simulink model "sg_2d_fir"  (Simulink 7.6)
settings: Solver=ode45  StartTime=0.0  StopTime=1600.0  RelTol=1e-3
undefined symbols (not defined in the file): gcbh, xlBlockLoadCallback, xlGetNormalizedPeriod, xlipgetpartsetting
libraries: xbsIndex_r4 x311, dspsrcs4 x6
(part 4 of 4)

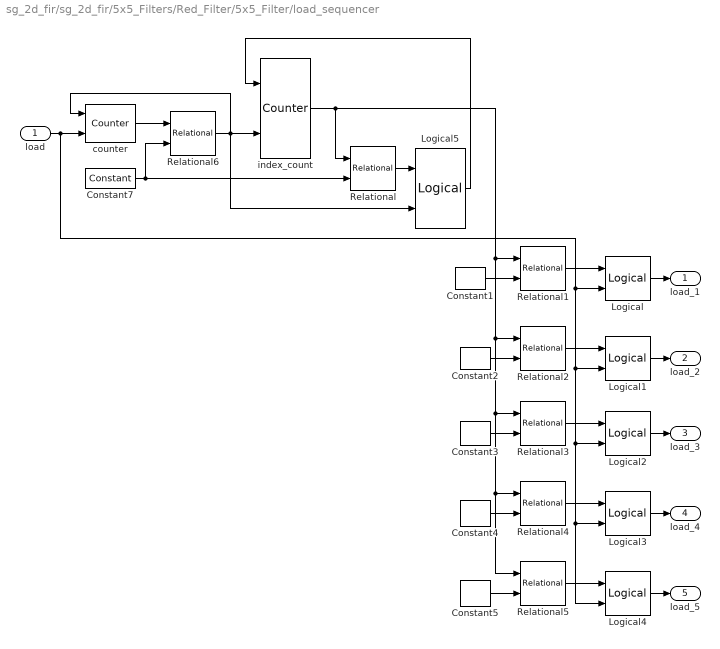
== system sg_2d_fir/sg_2d_fir/5x5_Filters/Red_Filter/5x5_Filter/load_sequencer ==
  load : Inport
  Constant1 : xbsIndex_r4/Constant  const=0  gui_display_data_type=Fixed-point  arith_type=Unsigned  n_bits=ceil(log2(num_coef))  bin_pt=0  preci_type=Single  exp_width=8  frac_width=24  explicit_period=off  period=1  equ=P=C  opselect=C  inp2=PCIN>>17  opr=+  inp1=P  carry=CIN  dbl_ovrd=off  block_type=constant
      settings: block_version=VER_STRING_GOES_HERE
  Constant2 : xbsIndex_r4/Constant  const=1  gui_display_data_type=Fixed-point  arith_type=Unsigned  n_bits=ceil(log2(num_coef))  bin_pt=0  preci_type=Single  exp_width=8  frac_width=24  explicit_period=off  period=1  equ=P=C  opselect=C  inp2=PCIN>>17  opr=+  inp1=P  carry=CIN  dbl_ovrd=off  block_type=constant
      settings: block_version=VER_STRING_GOES_HERE
  Constant3 : xbsIndex_r4/Constant  const=2  gui_display_data_type=Fixed-point  arith_type=Unsigned  n_bits=ceil(log2(num_coef))  bin_pt=0  preci_type=Single  exp_width=8  frac_width=24  explicit_period=off  period=1  equ=P=C  opselect=C  inp2=PCIN>>17  opr=+  inp1=P  carry=CIN  dbl_ovrd=off  block_type=constant
      settings: block_version=VER_STRING_GOES_HERE
  Constant4 : xbsIndex_r4/Constant  const=3  gui_display_data_type=Fixed-point  arith_type=Unsigned  n_bits=ceil(log2(num_coef))  bin_pt=0  preci_type=Single  exp_width=8  frac_width=24  explicit_period=off  period=1  equ=P=C  opselect=C  inp2=PCIN>>17  opr=+  inp1=P  carry=CIN  dbl_ovrd=off  block_type=constant
      settings: block_version=VER_STRING_GOES_HERE
  Constant5 : xbsIndex_r4/Constant  const=4  gui_display_data_type=Fixed-point  arith_type=Unsigned  n_bits=ceil(log2(num_coef))  bin_pt=0  preci_type=Single  exp_width=8  frac_width=24  explicit_period=off  period=1  equ=P=C  opselect=C  inp2=PCIN>>17  opr=+  inp1=P  carry=CIN  dbl_ovrd=off  block_type=constant
      settings: block_version=VER_STRING_GOES_HERE
  Constant7 : xbsIndex_r4/Constant  const=num_coef-1  gui_display_data_type=Fixed-point  arith_type=Unsigned  n_bits=ceil(log2(num_coef))  bin_pt=0  preci_type=Single  exp_width=8  frac_width=24  explicit_period=off  period=1  equ=P=C  opselect=C  inp2=PCIN>>17  opr=+  inp1=P  carry=CIN  dbl_ovrd=off  block_type=constant
      settings: block_version=VER_STRING_GOES_HERE
  Logical{,1..5} (6 alike) : xbsIndex_r4/Logical  logical_function=AND  inputs=2  en=off  latency=0  precision=Full  arith_type=Unsigned  n_bits=8  bin_pt=2  align_bp=on  dbl_ovrd=off  block_type=logical
      settings: xl_area=[0, 0, 0, 0, 0, 0, 0]  block_version=VER_STRING_GOES_HERE
  Relational{,1..6} (7 alike) : xbsIndex_r4/Relational  mode=a=b  en=off  latency=0  dbl_ovrd=off  block_type=relational
      settings: xl_area=[0, 0, 0, 0, 0, 0, 0]  block_version=VER_STRING_GOES_HERE
  counter : xbsIndex_r4/Counter  cnt_type=Count Limited  cnt_to=num_coef-1  operation=Up  start_count=0  cnt_by_val=1  arith_type=Unsigned  n_bits=ceil(log2(num_coef))  bin_pt=0  load_pin=off  rst=on  en=on  explicit_period=on  period=1  dbl_ovrd=off  use_behavioral_HDL=off  implementation=Fabric  use_rpm=off  block_type=counter
      settings: xl_area=[0, 0, 0, 0, 0, 0, 0]  block_version=VER_STRING_GOES_HERE
  index_count : xbsIndex_r4/Counter  cnt_type=Count Limited  cnt_to=num_coef-1  operation=Up  start_count=0  cnt_by_val=1  arith_type=Unsigned  n_bits=ceil(log2(num_coef))  bin_pt=0  load_pin=off  rst=on  en=on  explicit_period=on  period=1  dbl_ovrd=off  use_behavioral_HDL=off  implementation=Fabric  use_rpm=off  block_type=counter
      settings: infoedit="Configurable up, down and up/down counter.<P><P>Hardware notes: Free running counters are the least expensive in hardware.  A count limited counter is implemented by combining a counter with a comparator."  xl_area=[0, 0, 0, 0, 0, 0, 0]  block_version=VER_STRING_GOES_HERE
  load_1 : Outport
  load_2 : Outport  Port=2
  load_3 : Outport  Port=3
  load_4 : Outport  Port=4
  load_5 : Outport  Port=5
  wires:
  Constant1/1 -> Relational1/2
  Relational1/1 -> Logical/1
  Logical/1 -> load_1/1
  Constant2/1 -> Relational2/2
  Logical1/1 -> load_2/1
  Relational2/1 -> Logical1/1
  Constant3/1 -> Relational3/2
  Logical2/1 -> load_3/1
  Relational3/1 -> Logical2/1
  Constant4/1 -> Relational4/2
  Logical3/1 -> load_4/1
  Relational4/1 -> Logical3/1
  Constant5/1 -> Relational5/2
  Logical4/1 -> load_5/1
  Relational5/1 -> Logical4/1
  load/1 -> counter/2, Logical/2, Logical1/2, Logical2/2, Logical3/2, Logical4/2
  counter/1 -> Relational6/1
  Constant7/1 -> Relational6/2, Relational/2
  Relational6/1 -> index_count/2, counter/1, Logical5/2
  index_count/1 -> Relational/1, Relational1/1, Relational2/1, Relational3/1, Relational4/1, Relational5/1
  Relational/1 -> Logical5/1
  Logical5/1 -> index_count/1

== system sg_2d_fir/sg_2d_fir/5x5_Filters/Red_Filter/5x5_Filter/n-tap FIR Compiler Filter ==
  Din : Inport
  coef : Inport  Port=2
  load : Inport  Port=3
  "FIR Compiler 5.0 " : xbsIndex_r4/FIR Compiler 5.0   coefficientvector=coef  coefficient_sets=1  filter_type=Single_Rate  rate_change_type=Integer  interpolation_rate=1  decimation_rate=1  zero_pack_factor=1  number_channels=1  ratespecification=Maximum_Possible  sampleperiod=1  hardwareoversamplingrate=1  filter_architecture=Systolic_Multiply_Accumulate  coefficient_reload=on  coefficient_structure=Non_Symmetric  coefficient_sign=Signed  quantization=Quantize_Only  coefficient_width=coef_n_bits  bestprecision=off  coefficient_fractional_bits=coef_bin_pt  number_paths=1  output_rounding_mode=Full_Precision  output_width=26  allow_rounding_approximation=off  optimization_goal=Area  has_sclr=off  has_data_valid=off  has_nd=off  has_ce=off  usechan_in_adv=off  chan_in_adv=0  data_buffer_type=Automatic  coefficient_buffer_type=Automatic  input_buffer_type=Automatic  output_buffer_type=Automatic  preference_for_other_storage=Automatic  multi_column_support=Disabled  columnconfig='1'  inter_column_pipe_length=4  passband_min=0.0  passband_max=0.5  stopband_min=0.5  stopband_max=1.0  filter_selection=1  gui_behaviour=Sysgen  registered_output=true  data_sign=Signed  data_width=16  data_fractional_bits=0  wrapper_available=true  ip_wrap_arbitrary_binary_point=true  ip_name=FIR Compiler  ip_version=5.0  dsptool_ready=true  ipcore_usecache=true  ipcore_useipmodelcache=true  ipcore_xco_need_fpga_part=true  port_translation_map={ 'ce' => 'en', 'sclr' => 'rst' }  run_core_at_system_period=true  ipcore_fpga_part=xlipgetpartsetting(gcb, {'virtex4', 'xc4vsx35', '-10', 'ff668'})  structural_sim=false  block_type=fir_compiler_v5_0
      settings: block_version=11.2
  Register : xbsIndex_r4/Register  init=0  rst=off  en=on  dbl_ovrd=off  block_type=register
  Register2 : xbsIndex_r4/Register  init=0  rst=off  en=off  dbl_ovrd=off  block_type=register
      settings: block_version=9.1-beta
  Rising Edge Detector1 : Subsystem
  Terminator5 : Terminator
  Out : Outport
  wires:
  "FIR Compiler 5.0 "/2 -> Terminator5/1
  Rising Edge Detector1/1(Dout) -> "FIR Compiler 5.0 "/2
  Register2/1 -> "FIR Compiler 5.0 "/3
  load/1 -> Rising Edge Detector1/1(Din), Register2/1
  Register/1 -> Out/1
  coef/1 -> "FIR Compiler 5.0 "/4
  "FIR Compiler 5.0 "/1 -> Register/1
  "FIR Compiler 5.0 "/3 -> Register/2
  Din/1 -> "FIR Compiler 5.0 "/1

== system sg_2d_fir/sg_2d_fir/5x5_Filters/Red_Filter/5x5_Filter/n-tap FIR Compiler Filter1 ==
  Din : Inport
  coef : Inport  Port=2
  load : Inport  Port=3
  "FIR Compiler 5.0 " : xbsIndex_r4/FIR Compiler 5.0   coefficientvector=coef  coefficient_sets=1  filter_type=Single_Rate  rate_change_type=Integer  interpolation_rate=1  decimation_rate=1  zero_pack_factor=1  number_channels=1  ratespecification=Maximum_Possible  sampleperiod=1  hardwareoversamplingrate=1  filter_architecture=Systolic_Multiply_Accumulate  coefficient_reload=on  coefficient_structure=Non_Symmetric  coefficient_sign=Signed  quantization=Quantize_Only  coefficient_width=coef_n_bits  bestprecision=off  coefficient_fractional_bits=coef_bin_pt  number_paths=1  output_rounding_mode=Full_Precision  output_width=26  allow_rounding_approximation=off  optimization_goal=Area  has_sclr=off  has_data_valid=off  has_nd=off  has_ce=off  usechan_in_adv=off  chan_in_adv=0  data_buffer_type=Automatic  coefficient_buffer_type=Automatic  input_buffer_type=Automatic  output_buffer_type=Automatic  preference_for_other_storage=Automatic  multi_column_support=Disabled  columnconfig='1'  inter_column_pipe_length=4  passband_min=0.0  passband_max=0.5  stopband_min=0.5  stopband_max=1.0  filter_selection=1  gui_behaviour=Sysgen  registered_output=true  data_sign=Signed  data_width=16  data_fractional_bits=0  wrapper_available=true  ip_wrap_arbitrary_binary_point=true  ip_name=FIR Compiler  ip_version=5.0  dsptool_ready=true  ipcore_usecache=true  ipcore_useipmodelcache=true  ipcore_xco_need_fpga_part=true  port_translation_map={ 'ce' => 'en', 'sclr' => 'rst' }  run_core_at_system_period=true  ipcore_fpga_part=xlipgetpartsetting(gcb, {'virtex4', 'xc4vsx35', '-10', 'ff668'})  structural_sim=false  block_type=fir_compiler_v5_0
      settings: block_version=11.2
  Register : xbsIndex_r4/Register  init=0  rst=off  en=on  dbl_ovrd=off  block_type=register
  Register2 : xbsIndex_r4/Register  init=0  rst=off  en=off  dbl_ovrd=off  block_type=register
      settings: block_version=9.1-beta
  Rising Edge Detector1 : Subsystem
  Terminator5 : Terminator
  Out : Outport
  wires:
  Din/1 -> "FIR Compiler 5.0 "/1
  "FIR Compiler 5.0 "/3 -> Register/2
  "FIR Compiler 5.0 "/1 -> Register/1
  coef/1 -> "FIR Compiler 5.0 "/4
  Register/1 -> Out/1
  load/1 -> Register2/1, Rising Edge Detector1/1(Din)
  Register2/1 -> "FIR Compiler 5.0 "/3
  Rising Edge Detector1/1(Dout) -> "FIR Compiler 5.0 "/2
  "FIR Compiler 5.0 "/2 -> Terminator5/1

== system sg_2d_fir/sg_2d_fir/5x5_Filters/Red_Filter/5x5_Filter/n-tap FIR Compiler Filter2 ==
  Din : Inport
  coef : Inport  Port=2
  load : Inport  Port=3
  "FIR Compiler 5.0 " : xbsIndex_r4/FIR Compiler 5.0   coefficientvector=coef  coefficient_sets=1  filter_type=Single_Rate  rate_change_type=Integer  interpolation_rate=1  decimation_rate=1  zero_pack_factor=1  number_channels=1  ratespecification=Maximum_Possible  sampleperiod=1  hardwareoversamplingrate=1  filter_architecture=Systolic_Multiply_Accumulate  coefficient_reload=on  coefficient_structure=Non_Symmetric  coefficient_sign=Signed  quantization=Quantize_Only  coefficient_width=coef_n_bits  bestprecision=off  coefficient_fractional_bits=coef_bin_pt  number_paths=1  output_rounding_mode=Full_Precision  output_width=26  allow_rounding_approximation=off  optimization_goal=Area  has_sclr=off  has_data_valid=off  has_nd=off  has_ce=off  usechan_in_adv=off  chan_in_adv=0  data_buffer_type=Automatic  coefficient_buffer_type=Automatic  input_buffer_type=Automatic  output_buffer_type=Automatic  preference_for_other_storage=Automatic  multi_column_support=Disabled  columnconfig='1'  inter_column_pipe_length=4  passband_min=0.0  passband_max=0.5  stopband_min=0.5  stopband_max=1.0  filter_selection=1  gui_behaviour=Sysgen  registered_output=true  data_sign=Signed  data_width=16  data_fractional_bits=0  wrapper_available=true  ip_wrap_arbitrary_binary_point=true  ip_name=FIR Compiler  ip_version=5.0  dsptool_ready=true  ipcore_usecache=true  ipcore_useipmodelcache=true  ipcore_xco_need_fpga_part=true  port_translation_map={ 'ce' => 'en', 'sclr' => 'rst' }  run_core_at_system_period=true  ipcore_fpga_part=xlipgetpartsetting(gcb, {'virtex4', 'xc4vsx35', '-10', 'ff668'})  structural_sim=false  block_type=fir_compiler_v5_0
      settings: block_version=11.2
  Register : xbsIndex_r4/Register  init=0  rst=off  en=on  dbl_ovrd=off  block_type=register
  Register2 : xbsIndex_r4/Register  init=0  rst=off  en=off  dbl_ovrd=off  block_type=register
      settings: block_version=9.1-beta
  Rising Edge Detector1 : Subsystem
  Terminator5 : Terminator
  Out : Outport
  wires:
  "FIR Compiler 5.0 "/2 -> Terminator5/1
  Rising Edge Detector1/1(Dout) -> "FIR Compiler 5.0 "/2
  Register2/1 -> "FIR Compiler 5.0 "/3
  load/1 -> Rising Edge Detector1/1(Din), Register2/1
  Register/1 -> Out/1
  coef/1 -> "FIR Compiler 5.0 "/4
  "FIR Compiler 5.0 "/1 -> Register/1
  "FIR Compiler 5.0 "/3 -> Register/2
  Din/1 -> "FIR Compiler 5.0 "/1

== system sg_2d_fir/sg_2d_fir/5x5_Filters/Red_Filter/5x5_Filter/n-tap FIR Compiler Filter3 ==
  Din : Inport
  coef : Inport  Port=2
  load : Inport  Port=3
  "FIR Compiler 5.0 " : xbsIndex_r4/FIR Compiler 5.0   coefficientvector=coef  coefficient_sets=1  filter_type=Single_Rate  rate_change_type=Integer  interpolation_rate=1  decimation_rate=1  zero_pack_factor=1  number_channels=1  ratespecification=Maximum_Possible  sampleperiod=1  hardwareoversamplingrate=1  filter_architecture=Systolic_Multiply_Accumulate  coefficient_reload=on  coefficient_structure=Non_Symmetric  coefficient_sign=Signed  quantization=Quantize_Only  coefficient_width=coef_n_bits  bestprecision=off  coefficient_fractional_bits=coef_bin_pt  number_paths=1  output_rounding_mode=Full_Precision  output_width=26  allow_rounding_approximation=off  optimization_goal=Area  has_sclr=off  has_data_valid=off  has_nd=off  has_ce=off  usechan_in_adv=off  chan_in_adv=0  data_buffer_type=Automatic  coefficient_buffer_type=Automatic  input_buffer_type=Automatic  output_buffer_type=Automatic  preference_for_other_storage=Automatic  multi_column_support=Disabled  columnconfig='1'  inter_column_pipe_length=4  passband_min=0.0  passband_max=0.5  stopband_min=0.5  stopband_max=1.0  filter_selection=1  gui_behaviour=Sysgen  registered_output=true  data_sign=Signed  data_width=16  data_fractional_bits=0  wrapper_available=true  ip_wrap_arbitrary_binary_point=true  ip_name=FIR Compiler  ip_version=5.0  dsptool_ready=true  ipcore_usecache=true  ipcore_useipmodelcache=true  ipcore_xco_need_fpga_part=true  port_translation_map={ 'ce' => 'en', 'sclr' => 'rst' }  run_core_at_system_period=true  ipcore_fpga_part=xlipgetpartsetting(gcb, {'virtex4', 'xc4vsx35', '-10', 'ff668'})  structural_sim=false  block_type=fir_compiler_v5_0
      settings: block_version=11.2
  Register : xbsIndex_r4/Register  init=0  rst=off  en=on  dbl_ovrd=off  block_type=register
  Register2 : xbsIndex_r4/Register  init=0  rst=off  en=off  dbl_ovrd=off  block_type=register
      settings: block_version=9.1-beta
  Rising Edge Detector1 : Subsystem
  Terminator5 : Terminator
  Out : Outport
  wires:
  Din/1 -> "FIR Compiler 5.0 "/1
  "FIR Compiler 5.0 "/3 -> Register/2
  "FIR Compiler 5.0 "/1 -> Register/1
  coef/1 -> "FIR Compiler 5.0 "/4
  Register/1 -> Out/1
  load/1 -> Register2/1, Rising Edge Detector1/1(Din)
  Register2/1 -> "FIR Compiler 5.0 "/3
  Rising Edge Detector1/1(Dout) -> "FIR Compiler 5.0 "/2
  "FIR Compiler 5.0 "/2 -> Terminator5/1

== system sg_2d_fir/sg_2d_fir/5x5_Filters/Red_Filter/5x5_Filter/n-tap FIR Compiler Filter4 ==
  Din : Inport
  coef : Inport  Port=2
  load : Inport  Port=3
  "FIR Compiler 5.0 " : xbsIndex_r4/FIR Compiler 5.0   coefficientvector=coef  coefficient_sets=1  filter_type=Single_Rate  rate_change_type=Integer  interpolation_rate=1  decimation_rate=1  zero_pack_factor=1  number_channels=1  ratespecification=Maximum_Possible  sampleperiod=1  hardwareoversamplingrate=1  filter_architecture=Systolic_Multiply_Accumulate  coefficient_reload=on  coefficient_structure=Non_Symmetric  coefficient_sign=Signed  quantization=Quantize_Only  coefficient_width=coef_n_bits  bestprecision=off  coefficient_fractional_bits=coef_bin_pt  number_paths=1  output_rounding_mode=Full_Precision  output_width=26  allow_rounding_approximation=off  optimization_goal=Area  has_sclr=off  has_data_valid=off  has_nd=off  has_ce=off  usechan_in_adv=off  chan_in_adv=0  data_buffer_type=Automatic  coefficient_buffer_type=Automatic  input_buffer_type=Automatic  output_buffer_type=Automatic  preference_for_other_storage=Automatic  multi_column_support=Disabled  columnconfig='1'  inter_column_pipe_length=4  passband_min=0.0  passband_max=0.5  stopband_min=0.5  stopband_max=1.0  filter_selection=1  gui_behaviour=Sysgen  registered_output=true  data_sign=Signed  data_width=16  data_fractional_bits=0  wrapper_available=true  ip_wrap_arbitrary_binary_point=true  ip_name=FIR Compiler  ip_version=5.0  dsptool_ready=true  ipcore_usecache=true  ipcore_useipmodelcache=true  ipcore_xco_need_fpga_part=true  port_translation_map={ 'ce' => 'en', 'sclr' => 'rst' }  run_core_at_system_period=true  ipcore_fpga_part=xlipgetpartsetting(gcb, {'virtex4', 'xc4vsx35', '-10', 'ff668'})  structural_sim=false  block_type=fir_compiler_v5_0
      settings: block_version=11.2
  Register : xbsIndex_r4/Register  init=0  rst=off  en=on  dbl_ovrd=off  block_type=register
  Register2 : xbsIndex_r4/Register  init=0  rst=off  en=off  dbl_ovrd=off  block_type=register
      settings: block_version=9.1-beta
  Rising Edge Detector1 : Subsystem
  Terminator5 : Terminator
  Out : Outport
  wires:
  "FIR Compiler 5.0 "/2 -> Terminator5/1
  Rising Edge Detector1/1(Dout) -> "FIR Compiler 5.0 "/2
  Register2/1 -> "FIR Compiler 5.0 "/3
  load/1 -> Rising Edge Detector1/1(Din), Register2/1
  Register/1 -> Out/1
  coef/1 -> "FIR Compiler 5.0 "/4
  "FIR Compiler 5.0 "/1 -> Register/1
  "FIR Compiler 5.0 "/3 -> Register/2
  Din/1 -> "FIR Compiler 5.0 "/1

== system sg_2d_fir/sg_2d_fir/5x5_Filters/Blue_Filter/5x5_Filter/n-tap FIR Compiler Filter/Rising Edge Detector1 ==
  Din : Inport
  Inverter : xbsIndex_r4/Inverter  en=off  latency=0  dbl_ovrd=off  block_type=inv
      settings: block_version=9.1
  Logical : xbsIndex_r4/Logical  logical_function=AND  inputs=2  en=off  latency=0  precision=Full  arith_type=Unsigned  n_bits=16  bin_pt=0  align_bp=on  dbl_ovrd=off  block_type=logical
      settings: block_version=9.1
  Register1 : xbsIndex_r4/Register  init=0  rst=off  en=off  dbl_ovrd=off  block_type=register
      settings: block_version=9.1
  Dout : Outport
  wires:
  Logical/1 -> Dout/1
  Din/1 -> Register1/1, Logical/1
  Inverter/1 -> Logical/2
  Register1/1 -> Inverter/1

== system sg_2d_fir/sg_2d_fir/5x5_Filters/Blue_Filter/5x5_Filter/n-tap FIR Compiler Filter1/Rising Edge Detector1 ==
  Din : Inport
  Inverter : xbsIndex_r4/Inverter  en=off  latency=0  dbl_ovrd=off  block_type=inv
      settings: block_version=9.1
  Logical : xbsIndex_r4/Logical  logical_function=AND  inputs=2  en=off  latency=0  precision=Full  arith_type=Unsigned  n_bits=16  bin_pt=0  align_bp=on  dbl_ovrd=off  block_type=logical
      settings: block_version=9.1
  Register1 : xbsIndex_r4/Register  init=0  rst=off  en=off  dbl_ovrd=off  block_type=register
      settings: block_version=9.1
  Dout : Outport
  wires:
  Register1/1 -> Inverter/1
  Inverter/1 -> Logical/2
  Din/1 -> Logical/1, Register1/1
  Logical/1 -> Dout/1

== system sg_2d_fir/sg_2d_fir/5x5_Filters/Blue_Filter/5x5_Filter/n-tap FIR Compiler Filter2/Rising Edge Detector1 ==
  Din : Inport
  Inverter : xbsIndex_r4/Inverter  en=off  latency=0  dbl_ovrd=off  block_type=inv
      settings: block_version=9.1
  Logical : xbsIndex_r4/Logical  logical_function=AND  inputs=2  en=off  latency=0  precision=Full  arith_type=Unsigned  n_bits=16  bin_pt=0  align_bp=on  dbl_ovrd=off  block_type=logical
      settings: block_version=9.1
  Register1 : xbsIndex_r4/Register  init=0  rst=off  en=off  dbl_ovrd=off  block_type=register
      settings: block_version=9.1
  Dout : Outport
  wires:
  Logical/1 -> Dout/1
  Din/1 -> Register1/1, Logical/1
  Inverter/1 -> Logical/2
  Register1/1 -> Inverter/1

== system sg_2d_fir/sg_2d_fir/5x5_Filters/Blue_Filter/5x5_Filter/n-tap FIR Compiler Filter3/Rising Edge Detector1 ==
  Din : Inport
  Inverter : xbsIndex_r4/Inverter  en=off  latency=0  dbl_ovrd=off  block_type=inv
      settings: block_version=9.1
  Logical : xbsIndex_r4/Logical  logical_function=AND  inputs=2  en=off  latency=0  precision=Full  arith_type=Unsigned  n_bits=16  bin_pt=0  align_bp=on  dbl_ovrd=off  block_type=logical
      settings: block_version=9.1
  Register1 : xbsIndex_r4/Register  init=0  rst=off  en=off  dbl_ovrd=off  block_type=register
      settings: block_version=9.1
  Dout : Outport
  wires:
  Register1/1 -> Inverter/1
  Inverter/1 -> Logical/2
  Din/1 -> Logical/1, Register1/1
  Logical/1 -> Dout/1

== system sg_2d_fir/sg_2d_fir/5x5_Filters/Blue_Filter/5x5_Filter/n-tap FIR Compiler Filter4/Rising Edge Detector1 ==
  Din : Inport
  Inverter : xbsIndex_r4/Inverter  en=off  latency=0  dbl_ovrd=off  block_type=inv
      settings: block_version=9.1
  Logical : xbsIndex_r4/Logical  logical_function=AND  inputs=2  en=off  latency=0  precision=Full  arith_type=Unsigned  n_bits=16  bin_pt=0  align_bp=on  dbl_ovrd=off  block_type=logical
      settings: block_version=9.1
  Register1 : xbsIndex_r4/Register  init=0  rst=off  en=off  dbl_ovrd=off  block_type=register
      settings: block_version=9.1
  Dout : Outport
  wires:
  Logical/1 -> Dout/1
  Din/1 -> Register1/1, Logical/1
  Inverter/1 -> Logical/2
  Register1/1 -> Inverter/1

== system sg_2d_fir/sg_2d_fir/5x5_Filters/Green_Filter/5x5_Filter/n-tap FIR Compiler Filter/Rising Edge Detector1 ==
  Din : Inport
  Inverter : xbsIndex_r4/Inverter  en=off  latency=0  dbl_ovrd=off  block_type=inv
      settings: block_version=9.1
  Logical : xbsIndex_r4/Logical  logical_function=AND  inputs=2  en=off  latency=0  precision=Full  arith_type=Unsigned  n_bits=16  bin_pt=0  align_bp=on  dbl_ovrd=off  block_type=logical
      settings: block_version=9.1
  Register1 : xbsIndex_r4/Register  init=0  rst=off  en=off  dbl_ovrd=off  block_type=register
      settings: block_version=9.1
  Dout : Outport
  wires:
  Logical/1 -> Dout/1
  Din/1 -> Register1/1, Logical/1
  Inverter/1 -> Logical/2
  Register1/1 -> Inverter/1

== system sg_2d_fir/sg_2d_fir/5x5_Filters/Green_Filter/5x5_Filter/n-tap FIR Compiler Filter1/Rising Edge Detector1 ==
  Din : Inport
  Inverter : xbsIndex_r4/Inverter  en=off  latency=0  dbl_ovrd=off  block_type=inv
      settings: block_version=9.1
  Logical : xbsIndex_r4/Logical  logical_function=AND  inputs=2  en=off  latency=0  precision=Full  arith_type=Unsigned  n_bits=16  bin_pt=0  align_bp=on  dbl_ovrd=off  block_type=logical
      settings: block_version=9.1
  Register1 : xbsIndex_r4/Register  init=0  rst=off  en=off  dbl_ovrd=off  block_type=register
      settings: block_version=9.1
  Dout : Outport
  wires:
  Register1/1 -> Inverter/1
  Inverter/1 -> Logical/2
  Din/1 -> Logical/1, Register1/1
  Logical/1 -> Dout/1

== system sg_2d_fir/sg_2d_fir/5x5_Filters/Green_Filter/5x5_Filter/n-tap FIR Compiler Filter2/Rising Edge Detector1 ==
  Din : Inport
  Inverter : xbsIndex_r4/Inverter  en=off  latency=0  dbl_ovrd=off  block_type=inv
      settings: block_version=9.1
  Logical : xbsIndex_r4/Logical  logical_function=AND  inputs=2  en=off  latency=0  precision=Full  arith_type=Unsigned  n_bits=16  bin_pt=0  align_bp=on  dbl_ovrd=off  block_type=logical
      settings: block_version=9.1
  Register1 : xbsIndex_r4/Register  init=0  rst=off  en=off  dbl_ovrd=off  block_type=register
      settings: block_version=9.1
  Dout : Outport
  wires:
  Logical/1 -> Dout/1
  Din/1 -> Register1/1, Logical/1
  Inverter/1 -> Logical/2
  Register1/1 -> Inverter/1

== system sg_2d_fir/sg_2d_fir/5x5_Filters/Green_Filter/5x5_Filter/n-tap FIR Compiler Filter3/Rising Edge Detector1 ==
  Din : Inport
  Inverter : xbsIndex_r4/Inverter  en=off  latency=0  dbl_ovrd=off  block_type=inv
      settings: block_version=9.1
  Logical : xbsIndex_r4/Logical  logical_function=AND  inputs=2  en=off  latency=0  precision=Full  arith_type=Unsigned  n_bits=16  bin_pt=0  align_bp=on  dbl_ovrd=off  block_type=logical
      settings: block_version=9.1
  Register1 : xbsIndex_r4/Register  init=0  rst=off  en=off  dbl_ovrd=off  block_type=register
      settings: block_version=9.1
  Dout : Outport
  wires:
  Register1/1 -> Inverter/1
  Inverter/1 -> Logical/2
  Din/1 -> Logical/1, Register1/1
  Logical/1 -> Dout/1

== system sg_2d_fir/sg_2d_fir/5x5_Filters/Green_Filter/5x5_Filter/n-tap FIR Compiler Filter4/Rising Edge Detector1 ==
  Din : Inport
  Inverter : xbsIndex_r4/Inverter  en=off  latency=0  dbl_ovrd=off  block_type=inv
      settings: block_version=9.1
  Logical : xbsIndex_r4/Logical  logical_function=AND  inputs=2  en=off  latency=0  precision=Full  arith_type=Unsigned  n_bits=16  bin_pt=0  align_bp=on  dbl_ovrd=off  block_type=logical
      settings: block_version=9.1
  Register1 : xbsIndex_r4/Register  init=0  rst=off  en=off  dbl_ovrd=off  block_type=register
      settings: block_version=9.1
  Dout : Outport
  wires:
  Logical/1 -> Dout/1
  Din/1 -> Register1/1, Logical/1
  Inverter/1 -> Logical/2
  Register1/1 -> Inverter/1

== system sg_2d_fir/sg_2d_fir/5x5_Filters/Red_Filter/5x5_Filter/n-tap FIR Compiler Filter/Rising Edge Detector1 ==
  Din : Inport
  Inverter : xbsIndex_r4/Inverter  en=off  latency=0  dbl_ovrd=off  block_type=inv
      settings: block_version=9.1
  Logical : xbsIndex_r4/Logical  logical_function=AND  inputs=2  en=off  latency=0  precision=Full  arith_type=Unsigned  n_bits=16  bin_pt=0  align_bp=on  dbl_ovrd=off  block_type=logical
      settings: block_version=9.1
  Register1 : xbsIndex_r4/Register  init=0  rst=off  en=off  dbl_ovrd=off  block_type=register
      settings: block_version=9.1
  Dout : Outport
  wires:
  Register1/1 -> Inverter/1
  Inverter/1 -> Logical/2
  Din/1 -> Logical/1, Register1/1
  Logical/1 -> Dout/1

== system sg_2d_fir/sg_2d_fir/5x5_Filters/Red_Filter/5x5_Filter/n-tap FIR Compiler Filter1/Rising Edge Detector1 ==
  Din : Inport
  Inverter : xbsIndex_r4/Inverter  en=off  latency=0  dbl_ovrd=off  block_type=inv
      settings: block_version=9.1
  Logical : xbsIndex_r4/Logical  logical_function=AND  inputs=2  en=off  latency=0  precision=Full  arith_type=Unsigned  n_bits=16  bin_pt=0  align_bp=on  dbl_ovrd=off  block_type=logical
      settings: block_version=9.1
  Register1 : xbsIndex_r4/Register  init=0  rst=off  en=off  dbl_ovrd=off  block_type=register
      settings: block_version=9.1
  Dout : Outport
  wires:
  Logical/1 -> Dout/1
  Din/1 -> Register1/1, Logical/1
  Inverter/1 -> Logical/2
  Register1/1 -> Inverter/1

== system sg_2d_fir/sg_2d_fir/5x5_Filters/Red_Filter/5x5_Filter/n-tap FIR Compiler Filter2/Rising Edge Detector1 ==
  Din : Inport
  Inverter : xbsIndex_r4/Inverter  en=off  latency=0  dbl_ovrd=off  block_type=inv
      settings: block_version=9.1
  Logical : xbsIndex_r4/Logical  logical_function=AND  inputs=2  en=off  latency=0  precision=Full  arith_type=Unsigned  n_bits=16  bin_pt=0  align_bp=on  dbl_ovrd=off  block_type=logical
      settings: block_version=9.1
  Register1 : xbsIndex_r4/Register  init=0  rst=off  en=off  dbl_ovrd=off  block_type=register
      settings: block_version=9.1
  Dout : Outport
  wires:
  Register1/1 -> Inverter/1
  Inverter/1 -> Logical/2
  Din/1 -> Logical/1, Register1/1
  Logical/1 -> Dout/1

== system sg_2d_fir/sg_2d_fir/5x5_Filters/Red_Filter/5x5_Filter/n-tap FIR Compiler Filter3/Rising Edge Detector1 ==
  Din : Inport
  Inverter : xbsIndex_r4/Inverter  en=off  latency=0  dbl_ovrd=off  block_type=inv
      settings: block_version=9.1
  Logical : xbsIndex_r4/Logical  logical_function=AND  inputs=2  en=off  latency=0  precision=Full  arith_type=Unsigned  n_bits=16  bin_pt=0  align_bp=on  dbl_ovrd=off  block_type=logical
      settings: block_version=9.1
  Register1 : xbsIndex_r4/Register  init=0  rst=off  en=off  dbl_ovrd=off  block_type=register
      settings: block_version=9.1
  Dout : Outport
  wires:
  Logical/1 -> Dout/1
  Din/1 -> Register1/1, Logical/1
  Inverter/1 -> Logical/2
  Register1/1 -> Inverter/1

== system sg_2d_fir/sg_2d_fir/5x5_Filters/Red_Filter/5x5_Filter/n-tap FIR Compiler Filter4/Rising Edge Detector1 ==
  Din : Inport
  Inverter : xbsIndex_r4/Inverter  en=off  latency=0  dbl_ovrd=off  block_type=inv
      settings: block_version=9.1
  Logical : xbsIndex_r4/Logical  logical_function=AND  inputs=2  en=off  latency=0  precision=Full  arith_type=Unsigned  n_bits=16  bin_pt=0  align_bp=on  dbl_ovrd=off  block_type=logical
      settings: block_version=9.1
  Register1 : xbsIndex_r4/Register  init=0  rst=off  en=off  dbl_ovrd=off  block_type=register
      settings: block_version=9.1
  Dout : Outport
  wires:
  Register1/1 -> Inverter/1
  Inverter/1 -> Logical/2
  Din/1 -> Logical/1, Register1/1
  Logical/1 -> Dout/1
